simulink model "Carry_ripple_adder_8bit_Model"  (R2025a)
settings: Solver=VariableStepAuto  StartTime=0.0  StopTime=10.0  RelTol=1e-3
libraries: NSA_DEVS_SINKS x5, NSA_DEVS_DIGITALI3E_CONVERTER x3, NSA_DEVS_SOURCES x3, NSA_DEVS_DIGITALI3E_LOGIC x1
settings Model: Creator=david  LastModifiedBy=peter
settings RTWCC: GPUComputeCapability=3.5

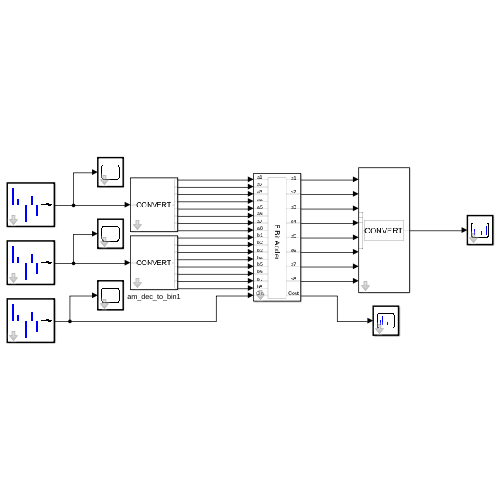
[thumbnail: Simulink's stored preview of the top-level diagram]
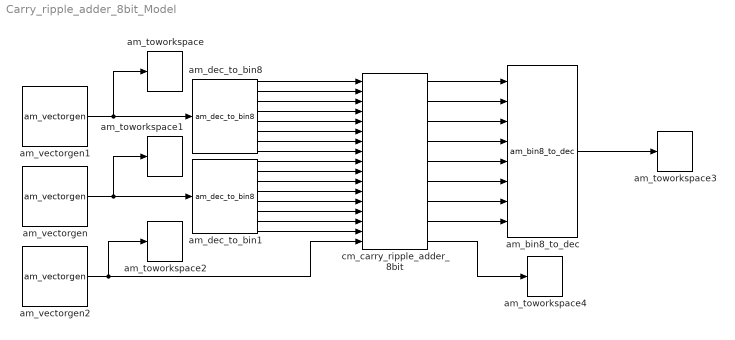
== system Carry_ripple_adder_8bit_Model ==
  am_bin8_to_dec : NSA_DEVS_DIGITALI3E_CONVERTER/am_bin8_to_dec  tau=[0,1]  debug=0
  am_dec_to_bin1 : NSA_DEVS_DIGITALI3E_CONVERTER/am_dec_to_bin8  tau=[0,1]  debug=0
  am_dec_to_bin8 : NSA_DEVS_DIGITALI3E_CONVERTER/am_dec_to_bin8  tau=[0,1]  debug=0
  am_toworkspace : NSA_DEVS_SINKS/am_toworkspace  varname="\"gen1Out\""  t0=0  format="\"vector\""  tau=[0,5]  debug=0
      settings: SourceProductName=Sinks
  am_toworkspace1 : NSA_DEVS_SINKS/am_toworkspace  varname="\"gen2Out\""  t0=0  format="\"vector\""  tau=[0,5]  debug=0
      settings: SourceProductName=Sinks
  am_toworkspace2 : NSA_DEVS_SINKS/am_toworkspace  varname="\"gen3Out\""  t0=0  format="\"vector\""  tau=[0,5]  debug=0
      settings: SourceProductName=Sinks
  am_toworkspace3 : NSA_DEVS_SINKS/am_toworkspace  varname="\"addersOut\""  t0=0  format="\"vector\""  tau=[0,5]  debug=0
      settings: SourceProductName=Sinks
  am_toworkspace4 : NSA_DEVS_SINKS/am_toworkspace  varname="\"addercOut\""  t0=0  format="\"vector\""  tau=[0,5]  debug=0
      settings: SourceProductName=Sinks
  am_vectorgen : NSA_DEVS_SOURCES/am_vectorgen  tvec=[1, 2, 3, 6]  yvec=[200, 240, 255, 100]  tau=[0,1]  debug=0
      settings: SourceProductName=Sources
  am_vectorgen1 : NSA_DEVS_SOURCES/am_vectorgen  tvec=[1, 4, 5, 6]  yvec=[10, 11, 12, 13]  tau=[0,1]  debug=0
      settings: SourceProductName=Sources
  am_vectorgen2 : NSA_DEVS_SOURCES/am_vectorgen  tvec=[1, 4, 5, 6]  yvec="[\"0\", \"1\", \"0\", \"0\"]"  tau=[0,1]  debug=0
      settings: SourceProductName=Sources
  cm_carry_ripple_adder_8bit : NSA_DEVS_DIGITALI3E_LOGIC/cm_carry_ripple_adder_8bit  tau=[0,1]  debug=0
  wires:
  am_dec_to_bin8/1 -> cm_carry_ripple_adder_8bit/1
  am_dec_to_bin8/2 -> cm_carry_ripple_adder_8bit/2
  am_dec_to_bin8/3 -> cm_carry_ripple_adder_8bit/3
  am_dec_to_bin8/4 -> cm_carry_ripple_adder_8bit/4
  am_dec_to_bin8/5 -> cm_carry_ripple_adder_8bit/5
  am_dec_to_bin8/6 -> cm_carry_ripple_adder_8bit/6
  am_dec_to_bin8/7 -> cm_carry_ripple_adder_8bit/7
  am_dec_to_bin8/8 -> cm_carry_ripple_adder_8bit/8
  am_dec_to_bin1/1 -> cm_carry_ripple_adder_8bit/9
  am_dec_to_bin1/2 -> cm_carry_ripple_adder_8bit/10
  am_dec_to_bin1/3 -> cm_carry_ripple_adder_8bit/11
  am_dec_to_bin1/4 -> cm_carry_ripple_adder_8bit/12
  am_dec_to_bin1/5 -> cm_carry_ripple_adder_8bit/13
  am_dec_to_bin1/6 -> cm_carry_ripple_adder_8bit/14
  am_dec_to_bin1/7 -> cm_carry_ripple_adder_8bit/15
  am_dec_to_bin1/8 -> cm_carry_ripple_adder_8bit/16
  am_vectorgen2/1 -> am_toworkspace2/1, cm_carry_ripple_adder_8bit/17
  cm_carry_ripple_adder_8bit/1 -> am_bin8_to_dec/1
  cm_carry_ripple_adder_8bit/2 -> am_bin8_to_dec/2
  cm_carry_ripple_adder_8bit/3 -> am_bin8_to_dec/3
  cm_carry_ripple_adder_8bit/4 -> am_bin8_to_dec/4
  cm_carry_ripple_adder_8bit/5 -> am_bin8_to_dec/5
  cm_carry_ripple_adder_8bit/6 -> am_bin8_to_dec/6
  cm_carry_ripple_adder_8bit/7 -> am_bin8_to_dec/7
  cm_carry_ripple_adder_8bit/8 -> am_bin8_to_dec/8
  am_bin8_to_dec/1 -> am_toworkspace3/1
  cm_carry_ripple_adder_8bit/9 -> am_toworkspace4/1
  am_vectorgen/1 -> am_toworkspace1/1, am_dec_to_bin1/1
  am_vectorgen1/1 -> am_toworkspace/1, am_dec_to_bin8/1
